simulink model "ImpedInvKin1"  (R2023b)
settings: Solver=VariableStepAuto  StartTime=0.0  StopTime=5  RelTol=1e-3
model workspace (MAT data in the model file):
  uini = Simulink.Parameter
  uini.DataType = 'auto'
  uini.Complexity = 'real'
  uini.Dimensions = [0 0]
  wn = 10
  zeta = 1
libraries: dspnetwork x2
settings Model: Creator=skala  LastModifiedBy=jeric
settings ModelReferenceCC: EnableRefExpFcnMdlSchedulingChecks=on

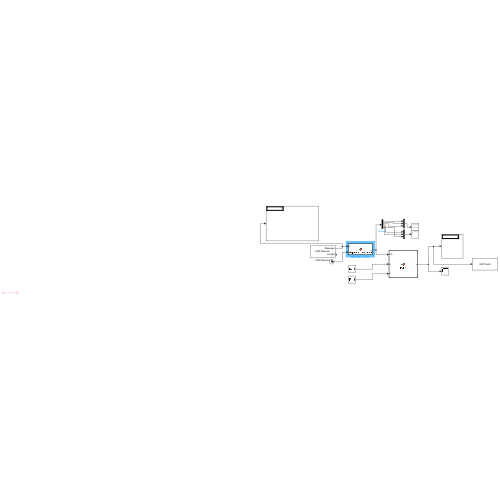
[thumbnail: Simulink's stored preview of the top-level diagram]
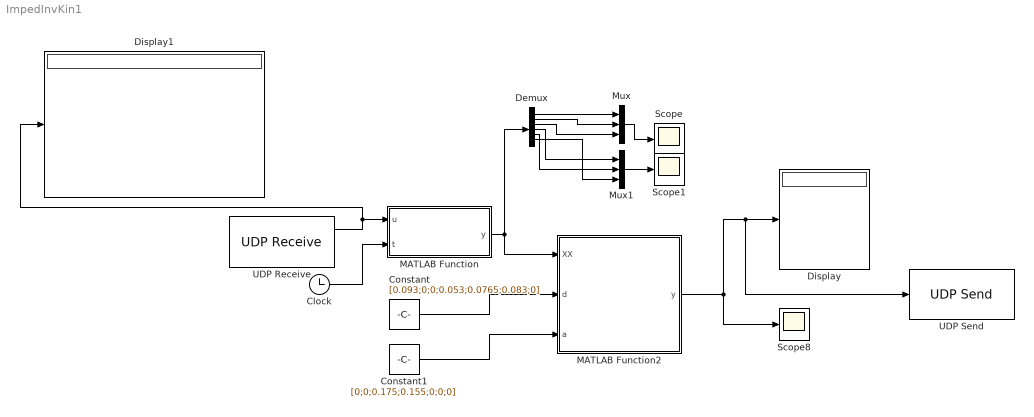
== system ImpedInvKin1 ==
  Clock : Clock
  Constant : Constant  Value=[0.093;0;0;0.053;0.0765;0.083;0]
  Constant1 : Constant  Value=[0;0;0.175;0.155;0;0;0]
  Demux : Demux  Outputs=6
  Display : Display
  Display1 : Display
  MATLAB Function : MATLAB Function  TreatAsAtomicUnit=on
  MATLAB Function2 : MATLAB Function  TreatAsAtomicUnit=on
  Mux : Mux  Inputs=3
  Mux1 : Mux  Inputs=3
  Scope : Scope
  Scope1 : Scope
  Scope8 : Scope
  UDP Receive : dspnetwork/UDP Receive  localURL='0.0.0.0'  localPort=25566  remoteURL='127.0.0.1'  remotePort=-1  recvBufferSize=2500  dims=24  signalDatatype=double  isComplex=off  isVarSize=off  showBlockingTime=off  blockingTime=0  sampletime=.0001  blockPlatform=[]
      settings: LibrarySourceBlock=dspsrcs4/UDP Receive
  UDP Send : dspnetwork/UDP Send  remoteURL='127.0.0.1'  remotePort=25565  localURL='0.0.0.0'  localPortSource=Automatically determine  localPort=-1  sendBufferSize=8192  sampletime=-1  blockPlatform=[]  separateLengthPort=0
      settings: LibrarySourceBlock=dspsnks4/UDP Send
  wires:
  MATLAB Function2/1(y) -> Display/1, UDP Send/1, Scope8/1
  ? -> ?
  UDP Receive/1 -> MATLAB Function/1(u), Display1/1
  Constant/1 -> MATLAB Function2/2(d)
  Constant1/1 -> MATLAB Function2/3(a)
  MATLAB Function/1(y) -> Demux/1, MATLAB Function2/1(XX)
  Demux/1 -> Mux/1
  Demux/2 -> Mux/2
  Demux/3 -> Mux/3
  Demux/4 -> Mux1/1
  Demux/5 -> Mux1/2
  Demux/6 -> Mux1/3
  Mux/1 -> Scope/1
  Mux1/1 -> Scope1/1
  Clock/1 -> MATLAB Function/2(t)

== matlab function ImpedInvKin1/MATLAB Function2 ==
  data: y output; XX input; d input; a input
function y= invkin(XX, d, a)
gamma=XX(1);beta=XX(2); alp=XX(3);
P=XX(4:6);
ROTg=[1 0 0; 0 cos(gamma) -sin(gamma); 0 sin(gamma) cos(gamma)];
ROTb=[cos(beta) 0 sin(beta); 0 1 0; -sin(beta) 0 cos(beta)];
ROTa=[cos(alp) -sin(alp) 0; sin(alp) cos(alp) 0; 0 0 1];
ROT=ROTa*ROTb*ROTg;
T07=[ROT P; 0 0 0 1];
d6=d(6); d4=d(4);
P6=T07(1:3,4);
k6=T07(1:3,3); m6=T07(1:3,1);
P5=P6-d6*k6;
x5=P5(1); y5=P5(2); 
mag5=sqrt(x5^2+y5^2);
theta1b=asin(d4/mag5)+atan2(y5,x5);
%%% ALTERNATIVE
%K1b=-y5; K2b=x5; K3b=d4;
%Topb=sqrt((K2b^2+K1b^2-K3b^2));
%Topb=sqrt((K2b^2+K1b^2-K3b^2));
%theta1b=2*atan((K2b-Topb)/(K3b+K1b));
%%%
r0=[sin(theta1b);-cos(theta1b);0];
u56=cross(r0,k6); u56m=sqrt(u56(1)^2+u56(2)^2+u56(3)^2);
v56m=dot(r0,k6);
theta5=atan2(u56m,v56m);
%%%%
%theta2i=ini(2); theta3i=ini(3); theta4i=ini(4);
%phi=theta2i+theta3i+theta4i-pi/2;
%%%% Calculation of phi
r1=[cos(theta1b);sin(theta1b);0];
k5=cross(r0,k6);
r11=cross(r1,k5); 
r12=dot(r1,k5);
mag11=sqrt(r11(1)^2+r11(2)^2+r11(3)^2);
phi=atan2(mag11,r12);
phi=acos(r12);
%%
a2=a(3); a3=a(4); d5=d(5); d1=d(1);
P5p=P5-d4*r0;
z5p=P5p(3); x5p=P5p(1); y5p=P5p(2);
xb=sqrt(x5p^2+y5p^2);
h=z5p-d1;
K1=2*a2*xb-2*a2*d5*cos(phi);
K2=2*a2*h-2*a2*d5*sin(phi);
K3=xb^2+h^2+a2^2+d5^2-a3^2-2*d5*h*sin(phi)-2*d5*xb*cos(phi);
Top=sqrt((K2^2+K1^2-K3^2));
theta2=2*atan((K2-Top)/(K3+K1));
%%%
K4=xb-a2*cos(theta2)-d5*cos(phi);
K5=a3*cos(theta2);
K6=a3*sin(theta2);
Top2=sqrt(K6^2+K5^2-K4^2);
theta3=2*atan((-K6+Top2)/(K4+K5));
theta4=phi-theta2-theta3+pi/2;
%%%
k5=[cos(phi)*cos(theta1b);cos(phi)*sin(theta1b);sin(phi)];
m5=cross(k6,k5);
%m6=T07(1:3,1);
xx=dot(m5,m6);
yyv=cross(m5,m6);
yy=sqrt(yyv(1)^2+yyv(2)^2+yyv(3)^2);
theta6a=atan2(yy,xx);
%theta6b=acos(xx);
%theta6=asin(yy);

y = [theta1b;theta2;theta3;theta4;theta5;theta6a]*180/pi;

== matlab function ImpedInvKin1/MATLAB Function ==
  data: u input; y output; t input
function y = TrajectoryGeneration(u, t)

tf = 5;
t0 = 0;

endEffector = u(16:21);
target = u(10:15);

A = [t0^5,   t0^4,    t0^3,    t0^2, t0, 1;
    5*t0^4,  4*t0^3,  3*t0^2,  2*t0, 1,  0;
    20*t0^3, 12*t0^2, 6*t0,    2,    0,  0;
    tf^5,    tf^4,    tf^3,    tf^2, tf, 1;
    5*tf^4,  4*tf^3,  3*tf^2,  2*tf, 1,  0;
    20*tf^3, 12*tf^2, 6*tf,    2,    0,  0;];

row1 = endEffector(1:6)';
row2 = target(1:6)';
B = [row1;
     0 0 0 0 0 0;
     0 0 0 0 0 0;
     row2;
     0 0 0 0 0 0;
     0 0 0 0 0 0;];

C = A \ B;

r = [t^5, t^4, t^3, t^2, t, 1];
position = [dot(r, C(1:6, 1));
            dot(r, C(1:6, 2));
            dot(r, C(1:6, 3));];

rotation = [dot(r, C(1:6, 4));
            dot(r, C(1:6, 5));
            dot(r, C(1:6, 6));];

y = [rotation; position];
